simulink model "IEEE39bus"  (Simulink 8.5)
settings: Solver=ode3  SolverMode=SingleTasking  StartTime=0.0  StopTime=50  FixedStep=Ts  RelTol=1e-3
PostLoadFcn:
  | Ts=25e-6; IEEE39BusLineLength;
  | vNomHV = 345E3;fNom=50;load('Dynamicload.mat');
InitFcn:
  | Ts=25e-6; IEEE39BusLineLength;
  | vNomHV = 345E3;fNom=50;load('Dynamicload.mat');
undefined symbols (not defined in the file): D1, Delta, load15, load16, load18, load20, load21, load23, load24, load25, load26, load27, load28, load29, load3, load39, load4, load7, load8, TL_10_11_len, TL_10_13_len, TL_13_14_len, TL_14_15_len, TL_15_16_len, TL_16_17_len, TL_16_19_len, TL_16_21_len, TL_16_24_len, TL_17_18_len, TL_17_27_len, TL_1_2_len, TL_1_39_len, TL_21_22_len, TL_22_23_len, TL_24_23_len, TL_25_26_len, TL_26_27_len, TL_26_28_len, TL_26_29_len, TL_28_29_len, TL_2_25_len, TL_2_2_len, TL_3_18_len, TL_3_4_len, TL_4_14_len, TL_4_5_len, TL_5_6_len, TL_5_8_len, TL_6_11_len, TL_6_7_len, TL_7_8_len, TL_8_9_len, TL_9_39_len
libraries: powerlib x175, op_dpl_lib x34, rtlab x14, sps_avr x9, powerlib_extras x2, artemis x1, powerlib_meascontrol x1
(part 1 of 5)
settings Model: ARTEMISmethode_block_infos=$$__separator__$$IEEE39bus/ARTEMIS Guide$$__separator__$$  Creator=Admin  LastModifiedBy=Administrator
settings OptimizationCC: BlockReduction=off  OptimizeBlockIOStorage=off  BufferReuse=off  GlobalBufferReuse=off  ExpressionFolding=off  LocalBlockOutputs=off
settings DebuggingCC: SolverPrmCheckMsg=warning  FcnCallInpInsideContextMsg=EnableAllAsWarning  UnconnectedInputMsg=none  UnconnectedOutputMsg=none  UnconnectedLineMsg=none

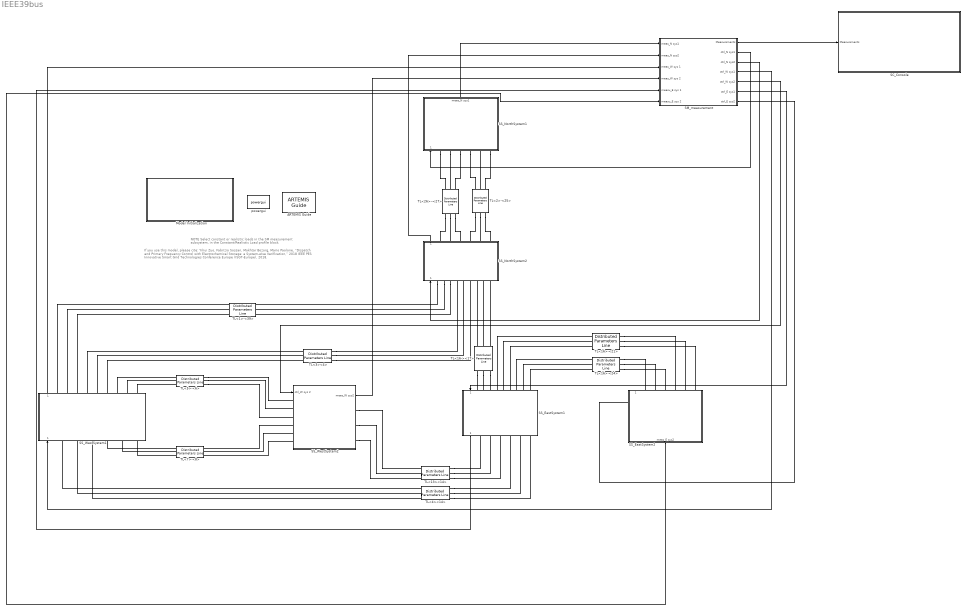
== system IEEE39bus ==
  note: If you use this model, please cite:
      | Yihui Zuo, Fabrizio Sossan, Mokhtar Bozorg, Mario Paolone,
      | “Dispatch and Primary Frequency Control with Electrochemical Storage: a System-wise Verification,”
      | 2018 IEEE PES Innovative Smart Grid Technologies Conference Europe (ISGT-Europe), 2018.
  note: NOTE
      | Select constant or realistic loads in the SM measurement
      | subsystem, in the Constant/Realistic Load profile block.
  ARTEMIS Guide : artemis/ARTEMIS/ARTEMIS Guide  Tag=FTSSmethode_opal_4hx0r99  Description=5.0_z1  lock=on  Ts=Ts  opt=art5  dyna=off  nb_perm=4  RT_fullcomp=off  ssn=on  ssn_itvc=off  ssn_ivic=off  ssn_ext=off  ssn_solver=Art5  ssn_impulse=off  ssn_quasimpulse=off  ssn_impulse_loop=2  paraExtinctionThy=off  Thy_Impulse=on  dtc=Off  dtc_opt=normal  ao=on  simtype=off  ct_mac=off  lin_mov=off  lsp=[0.001 2]  spike_skip=Disabled  dtc_extra=1  dtc_sws=normal  dtc_pied=0.5  SPSRulesBlock=SPSRules  tre=on  ctmm=off  LF=off  dpl_type=ARTEMiS DPL  rlc_type=off  custom_type=off  para=on  ssn_ImpulseLoopBlockedStateUpdate=2  ssn_mov_iter_number=5  ssn_switch_iter_number=5  ssn_nib_type_verify=on  ssn_use_lu=on  ssn_use_ldlt=off
  Model Initialization : Subsystem  AncestorBlock=artemis/Tools /Misc/Model Initialization  mask(Model Functions){InitFcnX=|, prel=off, posl=on, inif=on, strf=off}
      mask InitFcnX=|
      | Ts=25e-6; IEEE39BusLineLength;
      | vNomHV = 345E3;fNom=50;load('Dynamicload.mat');
      mask prompts: InitFcnX "Initialisation"; prel "Preload Function"; posl "PostLoad Function"; inif "InitFcn"; strf "StartFcn"
      mask init:
      | currentBlock = gcb;
      | root = bdroot(currentBlock);
      | 
      | if ~strcmp(get_param(root,'BlockDiagramType'),'library')
      |     if prel==1
      |         set_param(root, 'PreLoadFcn', InitFcnX);
      |     else
      |         set_param(root, 'PreLoadFcn', '');
      |     end
      |     if inif==1
      |         set_param(root, 'InitFcn', InitFcnX);
      |     else
      |         set_param(root, 'InitFcn', '');
      |     end
      |     if strf==1
      |         set_param(root, 'StartFcn', InitFcnX);
      |     else
      |         set_param(root, 'StartFcn', '');
      |     end
      |     if posl==1
      |         set_param(root, 'PostLoadFcn', InitFcnX);
      |     else
      |         set_param(root, 'PostLoadFcn', '');
      |     end
      | end
      | 
      | pos = get_param(currentBlock, 'Position');
      | width = pos(3) - pos(1); height = pos(4) - pos(2);
      | txt = [ upper(root) '\n' '- InitFcn. . . . . '  get_param(root, 'InitFcn') ];
      settings: CopyFcn=set_param(gcb,'LinkStatus','inactive')
      mask Display: text(5, height*0.5, txt, 'horizontalAlignment', 'left', 'verticalAlignment', 'middle') ;
  SC_Console : Subsystem
  SM_measurement : Subsystem
  SS_EastSystem1 : Subsystem
      mask Display: disp('Eastsystem 1')
  SS_EastSystem2 : Subsystem
      mask Display: disp('Eastsystem 2')
  SS_NorthSystem1 : Subsystem
      mask Display: disp('Northsystem 1')
  SS_NorthSystem2 : Subsystem
      mask Display: disp('Northsystem 2')
  SS_WestSystem1 : Subsystem
      mask Display: disp('WestSystem 1')
  SS_WestSystem2 : Subsystem
      mask Display: disp('Westsystem 2')
  TL<13><14> : op_dpl_lib/Distributed Parameters Line  SimulationMode=ARTEMIS model  Phases=3  Frequency=50  Resistance=[1.071 4.285]/TL_13_14_len  Inductance="[0.032  0.095]/TL_13_14_len"  Capacitance=[0.384e-6 0.175e-6]/TL_13_14_len  Length=TL_13_14_len  Measurements=None
  TL<16-><17> : op_dpl_lib/Distributed Parameters Line  SimulationMode=ARTEMIS model  Phases=3  Frequency=50  Resistance=[0.8332 3.33]/TL_16_17_len  Inductance="[0.028  0.084]/TL_16_17_len"  Capacitance=[0.299e-6 0.136e-6]/TL_16_17_len  Length=TL_16_17_len  Measurements=None
  TL<16>-<21> : op_dpl_lib/Distributed Parameters Line  SimulationMode=ARTEMIS model  Phases=3  Frequency=50  Resistance=[0.9522 3.809]/TL_16_21_len  Inductance="[0.043  0.128]/TL_16_21_len"  Capacitance=[0.568e-6 0.258e-6]/TL_16_21_len  Length=TL_16_21_len  Measurements=None
  TL<16>-<24> : op_dpl_lib/Distributed Parameters Line  SimulationMode=ARTEMIS model  Phases=3  Frequency=50  Resistance=[0.357 1.428]/TL_16_24_len  Inductance="[0.019  0.056]/TL_16_24_len"  Capacitance=[0.152e-6 0.069e-6]/TL_16_24_len  Length=TL_16_24_len  Measurements=None
  TL<1>-<39> : op_dpl_lib/Distributed Parameters Line  SimulationMode=ARTEMIS model  Phases=3  Frequency=50  Resistance=[1.19 4.76]/TL_1_39_len  Inductance="[0.079  0.237]/TL_1_39_len"  Capacitance=[1.67e-6 0.7599e-6]/TL_1_39_len  Length=TL_1_39_len  Measurements=None
  TL<26>--<27> : op_dpl_lib/Distributed Parameters Line  SimulationMode=ARTEMIS model  Phases=3  Frequency=50  Resistance=[1.666 6.665]/TL_26_27_len  Inductance="[0.046  0.139]/TL_26_27_len"  Capacitance=[0.534e-6 0.243e-6]/TL_26_27_len  Length=TL_26_27_len  Measurements=None
  TL<2>-<25> : op_dpl_lib/Distributed Parameters Line  SimulationMode=ARTEMIS model  Phases=3  Frequency=50  Resistance=[8.33 33.3]/TL_2_25_len  Inductance="[0.027  0.082]/TL_2_25_len"  Capacitance=[0.325e-6 0.148e-6]/TL_2_25_len  Length=TL_2_25_len  Measurements=None
  TL<3><4> : op_dpl_lib/Distributed Parameters Line  SimulationMode=ARTEMIS model  Phases=3  Frequency=50  Resistance=[1.547 6.18]/TL_3_4_len  Inductance="[0.067  0.208]/TL_3_4_len"  Capacitance=[0.493e-6 0.224e-6]/TL_3_4_len  Length=TL_3_4_len  Measurements=None
  TL<4><14> : op_dpl_lib/Distributed Parameters Line  SimulationMode=ARTEMIS model  Phases=3  Frequency=50  Resistance=[0.9522 3.808]/TL_4_14_len  Inductance="[0.041  0.1223]/TL_4_14_len"  Capacitance=[0.308e-6 0.14e-6]/TL_4_14_len  Length=TL_4_14_len  Measurements=None
  TL<5>-<6> : op_dpl_lib/Distributed Parameters Line  SimulationMode=ARTEMIS model  Phases=3  Frequency=50  Resistance=[0.476 1.904]/TL_5_6_len  Inductance=[0.014 0.04]/TL_5_6_len  Capacitance=[0.162e-6 0.074e-6]/TL_5_6_len  Length=TL_5_6_len  Measurements=None
  TL<7>-<8> : op_dpl_lib/Distributed Parameters Line  SimulationMode=ARTEMIS model  Phases=3  Frequency=50  Resistance=[0.476 1.904]/TL_7_8_len  Inductance="[0.015  0.044]/TL_7_8_len"  Capacitance=[0.174e-6 0.079e-6]/TL_7_8_len  Length=TL_7_8_len  Measurements=None
  powergui : powerlib/powergui  SimulationMode=Discrete  SolverType=Tustin  SampleTime=Ts  frequency=60  SPID=off  DisableSnubberDevices=off  DisableRonSwitches=off  DisableVfSwitches=off  SwTol=0  DisplayEquations=off  Interpol=off  methode=off  Ts=0  FunctionMessages=off  echomessages=off  HookPort=off  EnableUseOfTLC=off  x0status=steady  frequencyindice=0  Pbase=100e6  ErrMax=0.0001  Iterations=50  UnitsV=kV  UnitsW=MW  buscounter=0  RestoreLinks=warning  ResistiveCurrentMeasurement=off  Frange=[0:2:500]  Ylog=off  Xlog=on  ShowGrid=off  save=off  variable=ZData  structure=0  ZoomFFT=on  StartTime=0.0  cycles=1  DisplayStyle=1  fundamental=60  FreqAxis=off  MaxFrequency=1000  frequencyindicesteady=1  RmsSteady=2  display=off
  wires:
  SM_measurement/1(Measurements) -> SC_Console/1(Measurements)
  SM_measurement/5(ctrl_W sys2) -> SS_WestSystem2/1(ctrl_W sys 2)
  SM_measurement/6(ctrl_E sys1) -> SS_EastSystem1/1(ctrl_E sys1)
  SM_measurement/4(ctrl_W sys1) -> SS_WestSystem1/1(ctrl_W sys 1)
  SS_NorthSystem1/1(meas_N sys1) -> SM_measurement/1(meas_N sys1)
  SS_NorthSystem2/1(meas_N sys2) -> SM_measurement/2(" meas_N sys2")
  SS_EastSystem2/1(meas_E sys2) -> SM_measurement/6(measu_E sys 2)
  SS_EastSystem1/1(meas_E sys1) -> SM_measurement/5(measu_E sys 1)
  SS_WestSystem1/1(meas_W sys1) -> SM_measurement/3("meas_W sys 1  ")
  SS_WestSystem2/1(meas_W sys2) -> SM_measurement/4(" meas_W sys 2  ")
  SM_measurement/7(ctrl_E sys2) -> SS_EastSystem2/1(ctrl_E sys2)
  SM_measurement/3(ctrl_N sys2) -> SS_NorthSystem2/1(ctrl_N sys2)
  SM_measurement/2(ctrl_N sys1) -> SS_NorthSystem1/1(ctrl_N sys1)
  connections:
  SS_WestSystem1/RConn1 -- TL<1>-<39>/LConn1
  SS_WestSystem1/RConn2 -- TL<1>-<39>/LConn2
  SS_WestSystem1/RConn3 -- TL<1>-<39>/LConn3
  TL<3><4>/LConn1 -- SS_WestSystem1/RConn4
  TL<3><4>/LConn2 -- SS_WestSystem1/RConn5
  TL<3><4>/LConn3 -- SS_WestSystem1/RConn6
  TL<16-><17>/LConn2 -- SS_EastSystem1/LConn2
  TL<16-><17>/LConn1 -- SS_EastSystem1/LConn1
  TL<16-><17>/LConn3 -- SS_EastSystem1/LConn3
  TL<13><14>/RConn1 -- SS_EastSystem1/RConn1
  TL<13><14>/RConn2 -- SS_EastSystem1/RConn2
  TL<13><14>/RConn3 -- SS_EastSystem1/RConn3
  TL<4><14>/RConn1 -- SS_EastSystem1/RConn4
  TL<4><14>/RConn2 -- SS_EastSystem1/RConn5
  TL<4><14>/RConn3 -- SS_EastSystem1/RConn6
  SS_NorthSystem2/LConn1 -- TL<1>-<39>/RConn1
  SS_NorthSystem2/LConn2 -- TL<1>-<39>/RConn2
  SS_NorthSystem2/LConn3 -- TL<1>-<39>/RConn3
  TL<3><4>/RConn1 -- SS_NorthSystem2/LConn4
  TL<3><4>/RConn2 -- SS_NorthSystem2/LConn5
  TL<3><4>/RConn3 -- SS_NorthSystem2/LConn6
  TL<4><14>/LConn1 -- SS_WestSystem1/LConn1
  TL<4><14>/LConn2 -- SS_WestSystem1/LConn2
  TL<4><14>/LConn3 -- SS_WestSystem1/LConn3
  TL<16-><17>/RConn1 -- SS_NorthSystem2/LConn7
  TL<16-><17>/RConn2 -- SS_NorthSystem2/LConn8
  TL<16-><17>/RConn3 -- SS_NorthSystem2/LConn9
  SS_NorthSystem1/LConn2 -- TL<26>--<27>/LConn2
  TL<26>--<27>/RConn2 -- SS_NorthSystem2/RConn2
  TL<2>-<25>/LConn2 -- SS_NorthSystem1/LConn5
  TL<2>-<25>/RConn2 -- SS_NorthSystem2/RConn5
  SS_NorthSystem1/LConn6 -- TL<2>-<25>/LConn3
  SS_NorthSystem1/LConn4 -- TL<2>-<25>/LConn1
  SS_NorthSystem1/LConn3 -- TL<26>--<27>/LConn3
  SS_NorthSystem1/LConn1 -- TL<26>--<27>/LConn1
  TL<26>--<27>/RConn1 -- SS_NorthSystem2/RConn1
  TL<26>--<27>/RConn3 -- SS_NorthSystem2/RConn3
  TL<2>-<25>/RConn3 -- SS_NorthSystem2/RConn6
  TL<2>-<25>/RConn1 -- SS_NorthSystem2/RConn4
  TL<16>-<24>/LConn1 -- SS_EastSystem1/LConn7
  TL<16>-<24>/LConn2 -- SS_EastSystem1/LConn8
  TL<16>-<24>/LConn3 -- SS_EastSystem1/LConn9
  TL<16>-<24>/RConn3 -- SS_EastSystem2/LConn3
  TL<16>-<24>/RConn2 -- SS_EastSystem2/LConn2
  TL<16>-<24>/RConn1 -- SS_EastSystem2/LConn1
  SS_EastSystem1/LConn4 -- TL<16>-<21>/LConn1
  SS_EastSystem1/LConn5 -- TL<16>-<21>/LConn2
  SS_EastSystem1/LConn6 -- TL<16>-<21>/LConn3
  TL<16>-<21>/RConn1 -- SS_EastSystem2/LConn4
  TL<16>-<21>/RConn2 -- SS_EastSystem2/LConn5
  TL<16>-<21>/RConn3 -- SS_EastSystem2/LConn6
  SS_WestSystem2/RConn1 -- TL<13><14>/LConn1
  SS_WestSystem2/RConn2 -- TL<13><14>/LConn2
  SS_WestSystem2/RConn3 -- TL<13><14>/LConn3
  TL<5>-<6>/LConn1 -- SS_WestSystem1/RConn7
  TL<5>-<6>/LConn2 -- SS_WestSystem1/RConn8
  TL<5>-<6>/LConn3 -- SS_WestSystem1/RConn9
  TL<5>-<6>/RConn1 -- SS_WestSystem2/LConn1
  TL<5>-<6>/RConn2 -- SS_WestSystem2/LConn2
  TL<5>-<6>/RConn3 -- SS_WestSystem2/LConn3
  SS_WestSystem2/LConn4 -- TL<7>-<8>/RConn1
  SS_WestSystem2/LConn5 -- TL<7>-<8>/RConn2
  SS_WestSystem2/LConn6 -- TL<7>-<8>/RConn3
  TL<7>-<8>/LConn1 -- SS_WestSystem1/LConn4
  TL<7>-<8>/LConn2 -- SS_WestSystem1/LConn5
  TL<7>-<8>/LConn3 -- SS_WestSystem1/LConn6

== system IEEE39bus/Model Initialization ==

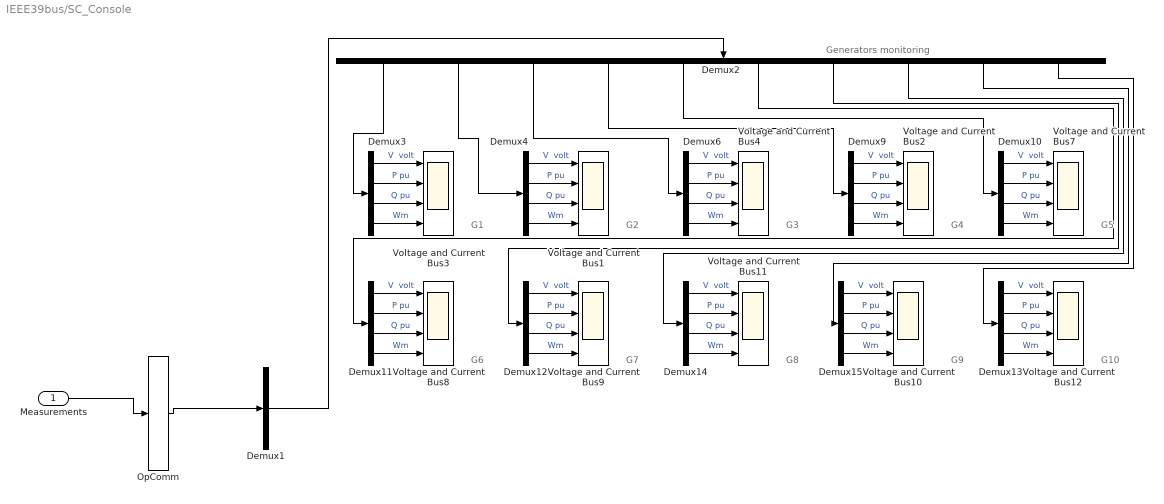
== system IEEE39bus/SC_Console ==
  note: G10
  note: G9
  note: G8
  note: G7
  note: G6
  note: G5
  note: G4
  note: G3
  note: G2
  note: G1
  note: Generators monitoring
  Measurements : Inport
  Demux1 : Demux  Outputs=[60 ]
  Demux{3..4,6,9..15} (10 alike) : Demux  Outputs=[3 1 1 1]
  Demux2 : Demux  Outputs=[6 6 6 6 6 6 6 6 6 6]
  OpComm : rtlab/OpComm  nbport=1  groupe_acq=1  subsys_rate=30*Ts  st=0  Synchronization=on  Interpolation=on  Threshold=1.0  Missed_Data=off  Sim_Time=off  Samples=off  dynSigOut=off  from_console=0  warning_done=off  writeOpCommFile=off  Offset=off
  Voltage and Current Bus{1..4,7..12} (10 alike) : Scope  NumInputPorts=4
      Voltage and Current Bus1 settings: TimeRange=0.24  YMin=-20000~0.715~0.2785~0.99755  YMax=20000~0.723~0.2835~0.99763  SaveName=mach  MaxDataPoints=15000
      Voltage and Current Bus10 settings: TimeRange=0.24  YMin=-20000~0.576~0.052~0.99807  YMax=20000~0.584~0.063~0.99816  SaveName=mach9  MaxDataPoints=15000
      Voltage and Current Bus11 settings: TimeRange=0.24  YMin=-20000~0.599~0.017~1.00427  YMax=20000~0.605~0.022~1.00438  SaveName=mach10  MaxDataPoints=15000
      Voltage and Current Bus12 settings: TimeRange=0.24  YMin=-20000~0.336~0.015~0.99933  YMax=20000~0.346~0.022~0.99942  SaveName=mach11  MaxDataPoints=15000
      Voltage and Current Bus2 settings: TimeRange=0.24  YMin=-20000~0.556~-0.038~0.99875  YMax=20000~0.563~-0.0335~0.99905  SaveName=mach2  MaxDataPoints=15000
      Voltage and Current Bus3 settings: TimeRange=22.5285  YMin=-20000~0.45~0.07~0.99775  YMax=20000~0.55~0.145~1.00125  SaveName=mach1  MaxDataPoints=15000
      Voltage and Current Bus4 settings: TimeRange=0.24  YMin=-20000~0.51~0.2~0.99932  YMax=20000~0.545~0.24~0.9994  SaveName=mach3  MaxDataPoints=15000
      Voltage and Current Bus7 settings: TimeRange=0.24  YMin=-20000~0.753~0.1225~0.982477  YMax=20000~0.7575~0.127~0.982495  SaveName=mach6  MaxDataPoints=15000
      Voltage and Current Bus8 settings: TimeRange=0.24  YMin=-20000~0.5~0.02~0.9963  YMax=20000~0.61~0.13~0.9973  SaveName=mach7  MaxDataPoints=15000
      Voltage and Current Bus9 settings: TimeRange=0.24  YMin=-20000~0.4425~-0.053~0.9993  YMax=20000~0.465~-0.046~0.99955  SaveName=mach8  MaxDataPoints=15000
  wires:
  Demux1/1 -> Demux2/1
  Demux2/10 -> Demux13/1
  Demux2/9 -> Demux15/1
  Demux2/8 -> Demux14/1
  Demux2/7 -> Demux12/1
  Demux2/6 -> Demux11/1
  Demux2/5 -> Demux10/1
  Demux2/4 -> Demux9/1
  Demux2/3 -> Demux6/1
  Demux2/2 -> Demux4/1
  Demux2/1 -> Demux3/1
  OpComm/1 -> Demux1/1
  Measurements/1 -> OpComm/1
  Demux3/1 -> Voltage and Current Bus3/1  "V  volt"
  Demux3/3 -> Voltage and Current Bus3/3  "Q pu"
  Demux3/4 -> Voltage and Current Bus3/4  "Wm"
  Demux3/2 -> Voltage and Current Bus3/2  "P pu"
  Demux4/1 -> Voltage and Current Bus1/1  "V  volt"
  Demux4/3 -> Voltage and Current Bus1/3  "Q pu"
  Demux4/4 -> Voltage and Current Bus1/4  "Wm"
  Demux4/2 -> Voltage and Current Bus1/2  "P pu"
  Demux6/1 -> Voltage and Current Bus4/1  "V  volt"
  Demux6/3 -> Voltage and Current Bus4/3  "Q pu"
  Demux6/4 -> Voltage and Current Bus4/4  "Wm"
  Demux6/2 -> Voltage and Current Bus4/2  "P pu"
  Demux9/1 -> Voltage and Current Bus2/1  "V  volt"
  Demux9/3 -> Voltage and Current Bus2/3  "Q pu"
  Demux9/4 -> Voltage and Current Bus2/4  "Wm"
  Demux9/2 -> Voltage and Current Bus2/2  "P pu"
  Demux10/1 -> Voltage and Current Bus7/1  "V  volt"
  Demux10/3 -> Voltage and Current Bus7/3  "Q pu"
  Demux10/4 -> Voltage and Current Bus7/4  "Wm"
  Demux10/2 -> Voltage and Current Bus7/2  "P pu"
  Demux11/1 -> Voltage and Current Bus8/1  "V  volt"
  Demux11/3 -> Voltage and Current Bus8/3  "Q pu"
  Demux11/4 -> Voltage and Current Bus8/4  "Wm"
  Demux11/2 -> Voltage and Current Bus8/2  "P pu"
  Demux12/1 -> Voltage and Current Bus9/1  "V  volt"
  Demux12/3 -> Voltage and Current Bus9/3  "Q pu"
  Demux12/4 -> Voltage and Current Bus9/4  "Wm"
  Demux12/2 -> Voltage and Current Bus9/2  "P pu"
  Demux14/1 -> Voltage and Current Bus11/1  "V  volt"
  Demux14/3 -> Voltage and Current Bus11/3  "Q pu"
  Demux14/4 -> Voltage and Current Bus11/4  "Wm"
  Demux14/2 -> Voltage and Current Bus11/2  "P pu"
  Demux15/1 -> Voltage and Current Bus10/1  "V  volt"
  Demux15/3 -> Voltage and Current Bus10/3  "Q pu"
  Demux15/4 -> Voltage and Current Bus10/4  "Wm"
  Demux15/2 -> Voltage and Current Bus10/2  "P pu"
  Demux13/1 -> Voltage and Current Bus12/1  "V  volt"
  Demux13/3 -> Voltage and Current Bus12/3  "Q pu"
  Demux13/4 -> Voltage and Current Bus12/4  "Wm"
  Demux13/2 -> Voltage and Current Bus12/2  "P pu"

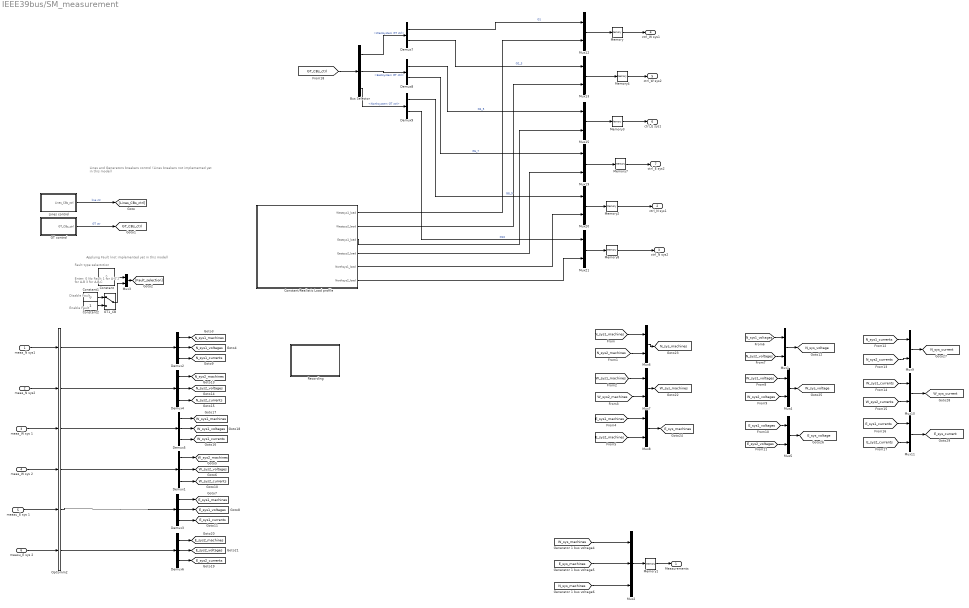
== system IEEE39bus/SM_measurement ==
  note: Enable Fault
  note: Disable Fault
  note: Enter:  0 No Fault
      |          1 for A-G
      |          2 for A-B
      |              3 for A-B-C
  note: Fault type selectction
  note: Applying Fault
      | (not implemented yet in this model)
  note: Lines and Generators breakers control
      | (Lines breakers not implemented yet in this model)
  meas_N sys1 : Inport
  " meas_N sys2" : Inport  Port=2
  "meas_W sys 1  " : Inport  Port=3
  " meas_W sys 2  " : Inport  Port=4
  measu_E sys 1 : Inport  Port=5
  measu_E sys 2 : Inport  Port=6
  Bus Selector : BusSelector  OutputSignals=Westsystem GT ctrl,Eastsystem GT ctrl,Northsystem GT ctrl
  Constant : Constant  Value=2
  Constant/Realistic Load profile : Subsystem  SystemSampleTime=20e-3  mask{Loadselect=Constant Load}
      mask init:
      | if (Loadselect == 1)
      |     mode = 0;
      | else 
      |         mode = 1; 
      | end
      mask TypeOptions Loadselect: Constant Load | Realistic Load
      mask Display: disp('Load Profile \n Constant / Realistic')
  Constant1 : Constant  Value=0
  Constant2 : Constant
  Demux1 : Demux  Outputs=[12 18 18]
  Demux2 : Demux  Outputs=[12 12 12]
  Demux3 : Demux  Outputs=[12 15 15]
  Demux4 : Demux  Outputs=[6 18 18]
  Demux5 : Demux  Outputs=[6 15 15]
  Demux6 : Demux  Outputs=[12 12 12]
  Demux7 : Demux  Outputs=[1 2]
  Demux8 : Demux  Outputs=[2 2]
  Demux9 : Demux  Outputs=[2 1]
  GT control : Subsystem
  GT1_CB : ManualSwitch
  Lines control : Subsystem
  Memory{,1..4,7..8} (7 alike) : Memory
  Mux{1,3..13,15,19..21} (16 alike) : Mux  Inputs=2
  Mux2 : Mux  Inputs=3
  OpComm2 : rtlab/OpComm  nbport=6  groupe_acq=1  subsys_rate=0  st=Ts  Synchronization=on  Interpolation=on  Threshold=1.0  Missed_Data=off  Sim_Time=off  Samples=off  dynSigOut=off  from_console=0  warning_done=off  writeOpCommFile=off  Offset=off
  Recording : Subsystem
  Measurements : Outport
  ctrl_N sys1 : Outport  Port=2
  ctrl_N sys2 : Outport  Port=3
  ctrl_W sys1 : Outport  Port=4
  ctrl_W sys2 : Outport  Port=5
  ctrl_E sys1 : Outport  Port=6
  ctrl_E sys2 : Outport  Port=7
  tag scope: E_sys1_currents=global, E_sys1_machines=global, E_sys1_voltages=global, E_sys2_currents=global, E_sys2_machines=global, E_sys2_voltages=global, E_sys_current=global, E_sys_machines=global, E_sys_voltage=global, GT_CBs_ctrl=global, N_sys1_currents=global, N_sys1_machines=global, N_sys1_voltages=global, N_sys2_currents=global, N_sys2_machines=global, N_sys2_voltages=global, N_sys_current=global, N_sys_machines=global, N_sys_voltage=global, W_sys1_currents=global, W_sys1_machines=global, W_sys1_voltages=global, W_sys2_currents=global, W_sys2_machines=global, W_sys2_voltages=global, W_sys_current=global, W_sys_machines=global, W_sys_voltage=global
  wires:
  Demux3/2 -> [E_sys1_voltages]
  Demux1/2 -> [W_sys2_voltages]
  Demux2/2 -> [N_sys1_voltages]
  Memory1/1 -> Measurements/1
  [N_sys_machines] -> Mux2/3
  [E_sys_machines] -> Mux2/2
  [W_sys_machines] -> Mux2/1
  Demux3/1 -> [E_sys1_machines]
  Demux1/1 -> [W_sys2_machines]
  " meas_W sys 2  "/1 -> OpComm2/4
  " meas_N sys2"/1 -> OpComm2/2
  Mux2/1 -> Memory1/1
  OpComm2/1 -> Demux2/1
  Demux2/1 -> [N_sys1_machines]
  Demux2/3 -> [N_sys1_currents]
  Demux1/3 -> [W_sys2_currents]
  Demux3/3 -> [E_sys1_currents]
  Constant/1 -> Mux3/1
  GT1_CB/1 -> Mux3/2
  Constant1/1 -> GT1_CB/1
  Constant2/1 -> GT1_CB/2
  GT control/1(GT_CBs_ctrl) -> [GT_CBs_ctrl]  "GT ctr"
  Lines control/1(Lines_CBs_ctrl) -> [Lines_CBs_ctrl]  "line ctr"
  Mux3/1 -> [Fault_selection]
  meas_N sys1/1 -> OpComm2/1
  "meas_W sys 1  "/1 -> OpComm2/3
  measu_E sys 1/1 -> OpComm2/5
  measu_E sys 2/1 -> OpComm2/6
  Demux4/2 -> [N_sys2_voltages]
  Demux4/1 -> [N_sys2_machines]
  Demux4/3 -> [N_sys2_currents]
  OpComm2/2 -> Demux4/1
  OpComm2/4 -> Demux1/1
  Demux5/2 -> [W_sys1_voltages]
  Demux5/1 -> [W_sys1_machines]
  Demux5/3 -> [W_sys1_currents]
  OpComm2/3 -> Demux5/1
  OpComm2/5 -> Demux3/1
  Demux6/2 -> [E_sys2_voltages]
  Demux6/1 -> [E_sys2_machines]
  Demux6/3 -> [E_sys2_currents]
  OpComm2/6 -> Demux6/1
  [N_sys2_machines] -> Mux6/2
  [N_sys1_machines] -> Mux6/1
  Mux6/1 -> [N_sys_machines]
  [W_sys1_machines] -> Mux7/1
  [W_sys2_machines] -> Mux7/2
  Mux7/1 -> [W_sys_machines]
  [E_sys1_machines] -> Mux8/1
  [E_sys2_machines] -> Mux8/2
  Mux8/1 -> [E_sys_machines]
  [N_sys1_voltages] -> Mux1/1
  [N_sys2_voltages] -> Mux1/2
  [W_sys1_voltages] -> Mux4/1
  [W_sys2_voltages] -> Mux4/2
  [E_sys1_voltages] -> Mux5/1
  [E_sys2_voltages] -> Mux5/2
  Mux1/1 -> [N_sys_voltage]
  Mux4/1 -> [W_sys_voltage]
  Mux5/1 -> [E_sys_voltage]
  [N_sys1_currents] -> Mux9/1
  [N_sys2_currents] -> Mux9/2
  [W_sys1_currents] -> Mux10/1
  [W_sys2_currents] -> Mux10/2
  [E_sys1_currents] -> Mux11/1
  [E_sys2_currents] -> Mux11/2
  Mux9/1 -> [N_sys_current]
  Mux10/1 -> [W_sys_current]
  Mux11/1 -> [E_sys_current]
  Memory2/1 -> ctrl_N sys1/1
  Memory3/1 -> ctrl_E sys1/1
  Memory/1 -> ctrl_W sys1/1
  Constant/Realistic Load profile/1(Westsys1_load) -> Mux12/2
  Constant/Realistic Load profile/2(Westsys2_laod) -> Mux13/2
  Memory4/1 -> ctrl_W sys2/1
  Constant/Realistic Load profile/3(Eastsys1_load) -> Mux15/2
  Constant/Realistic Load profile/4(Eastsys2_load) -> Mux19/2
  Memory7/1 -> ctrl_E sys2/1
  Constant/Realistic Load profile/5(Northsys1_load) -> Mux20/2
  Constant/Realistic Load profile/6(Northsys2_load) -> Mux21/2
  Memory8/1 -> ctrl_N sys2/1
  Mux20/1 -> Memory2/1
  [GT_CBs_ctrl] -> Bus Selector/1
  Bus Selector/2 -> Demux8/1  "<Eastsystem GT ctrl>"
  Bus Selector/1 -> Demux7/1  "<Westsystem GT ctrl>"
  Bus Selector/3 -> Demux9/1  "<Northsystem GT ctrl>"
  Demux7/1 -> Mux12/1  "G1"
  Mux12/1 -> Memory/1
  Demux7/2 -> Mux13/1  "G2_3"
  Mux13/1 -> Memory4/1
  Demux8/1 -> Mux15/1  "G4_5"
  Demux8/2 -> Mux19/1  "G6_7"
  Mux15/1 -> Memory3/1
  Mux19/1 -> Memory7/1
  Demux9/1 -> Mux20/1  "G8_9"
  Demux9/2 -> Mux21/1  "G10"
  Mux21/1 -> Memory8/1

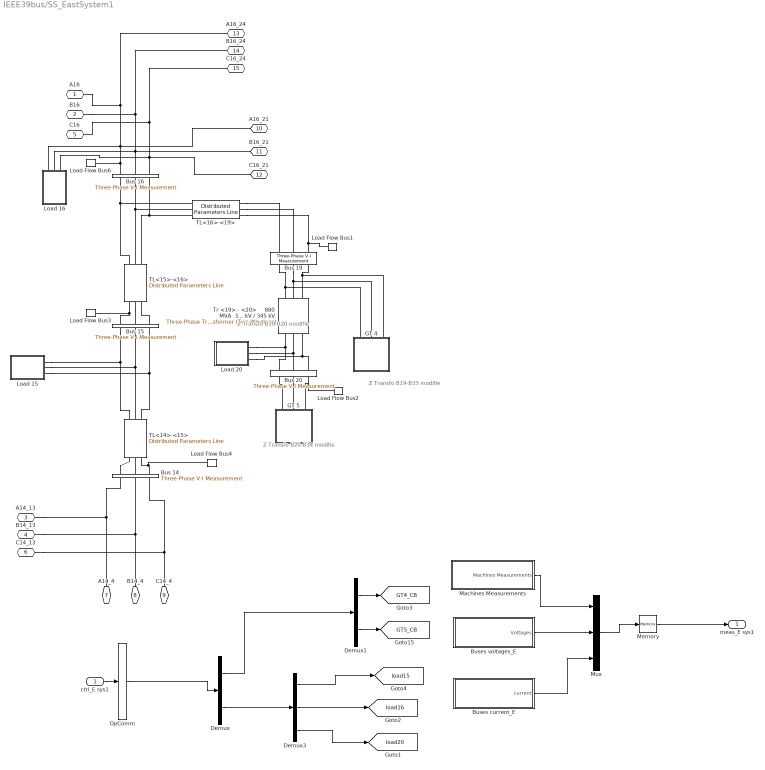
== system IEEE39bus/SS_EastSystem1 ==
  note: Z Transfo B19-B20 modifie
  note: Z Transfo B20-B34 modifie
  note: Z Transfo B19-B33 modifie
  ctrl_E sys1 : Inport
  Bus 14 : powerlib/Measurements/Three-Phase V-I Measurement  VoltageMeasurement=phase-to-ground  SetLabelV=on  LabelV=V_bus_14  Vpu=off  VpuLL=off  CurrentMeasurement=yes  SetLabelI=on  LabelI=I_bus_14  Ipu=off  Pbase=100e6  Vbase=230e3  OutputType=Complex  PhasorSimulation=off  PSBequivalent=0
  Bus 15 : powerlib/Measurements/Three-Phase V-I Measurement  VoltageMeasurement=phase-to-ground  SetLabelV=on  LabelV=V_bus_15  Vpu=off  VpuLL=off  CurrentMeasurement=yes  SetLabelI=on  LabelI=I_bus_15  Ipu=off  Pbase=100e6  Vbase=230e3  OutputType=Complex  PhasorSimulation=off  PSBequivalent=0
  Bus 16 : powerlib/Measurements/Three-Phase V-I Measurement  VoltageMeasurement=phase-to-ground  SetLabelV=on  LabelV=V_bus_16  Vpu=off  VpuLL=off  CurrentMeasurement=yes  SetLabelI=on  LabelI=I_bus_16  Ipu=off  Pbase=100e6  Vbase=230e3  OutputType=Complex  PhasorSimulation=off  PSBequivalent=0
  Bus 19 : powerlib/Measurements/Three-Phase V-I Measurement  VoltageMeasurement=phase-to-ground  SetLabelV=on  LabelV=V_bus_19  Vpu=off  VpuLL=off  CurrentMeasurement=yes  SetLabelI=on  LabelI=I_bus_19  Ipu=off  Pbase=100e6  Vbase=230e3  OutputType=Complex  PhasorSimulation=off  PSBequivalent=0
  Bus 20 : powerlib/Measurements/Three-Phase V-I Measurement  VoltageMeasurement=phase-to-ground  SetLabelV=on  LabelV=V_bus_20  Vpu=off  VpuLL=off  CurrentMeasurement=yes  SetLabelI=on  LabelI=I_bus_20  Ipu=off  Pbase=100e6  Vbase=230e3  OutputType=Complex  PhasorSimulation=off  PSBequivalent=0
  Buses current_E : Subsystem
  Buses voltages_E : Subsystem
  Demux : Demux  Outputs=[2 6]
  Demux1 : Demux  Outputs=2
  Demux3 : Demux  Outputs=[2 2 2]
  GT 4 : Subsystem
  GT 5 : Subsystem
  Load 15 : Subsystem
  Load 16 : Subsystem
  Load 20 : Subsystem
  Load Flow Bus1 : powerlib/Measurements/Load Flow Bus  LConnTagsString=a  ID=Bus-19  Vbase=345e+003  Vref=1  Vangle=0  VLF=1.019  angleLF=21.55
      settings: AttributesFormatString=%<ID>\n%<Vbase>V\n%<VLF>pu\n%<angleLF>deg.
  Load Flow Bus2 : powerlib/Measurements/Load Flow Bus  LConnTagsString=a  ID=Bus-20  Vbase=345e+003  Vref=1  Vangle=0  VLF=0.9613  angleLF=-10.55
      settings: AttributesFormatString=%<ID>\n%<Vbase>V\n%<VLF>pu\n%<angleLF>deg.
  Load Flow Bus3 : powerlib/Measurements/Load Flow Bus  LConnTagsString=a  ID=Bus-15  Vbase=345e+003  Vref=1  Vangle=0  VLF=0.996  angleLF=18.53
      settings: AttributesFormatString=%<ID>\n%<Vbase>V\n%<VLF>pu\n%<angleLF>deg.
  Load Flow Bus4 : powerlib/Measurements/Load Flow Bus  LConnTagsString=a  ID=Bus-14  Vbase=345e+003  Vref=1  Vangle=0  VLF=1.001  angleLF=20.12
      settings: AttributesFormatString=%<ID>\n%<Vbase>V\n%<VLF>pu\n%<angleLF>deg.
  Load Flow Bus6 : powerlib/Measurements/Load Flow Bus  LConnTagsString=a  ID=Bus-16  Vbase=345e+003  Vref=1  Vangle=0  VLF=1.007  angleLF=19.22
      settings: AttributesFormatString=%<ID>\n%<Vbase>V\n%<VLF>pu\n%<angleLF>deg.
  Machines Measurements : Subsystem
      mask Display: disp('Machines Measurements')
  Memory : Memory
  Mux : Mux  Inputs=3
  OpComm : rtlab/OpComm  nbport=1  groupe_acq=1  subsys_rate=0  st=0  Synchronization=on  Interpolation=on  Threshold=1.0  Missed_Data=off  Sim_Time=off  Samples=off  dynSigOut=off  from_console=0  warning_done=off  writeOpCommFile=off  Offset=off
  TL<14>-<15> : op_dpl_lib/Distributed Parameters Line  SimulationMode=ARTEMIS model  Phases=3  Frequency=50  Resistance=[2.142 8.57]/TL_14_15_len  Inductance="[0.069  0.206]/TL_14_15_len"  Capacitance=[0.816e-6 0.371e-6]/TL_14_15_len  Length=TL_14_15_len  Measurements=None
  TL<15>-<16> : op_dpl_lib/Distributed Parameters Line  SimulationMode=ARTEMIS model  Phases=3  Frequency=50  Resistance=[1.071 4.285]/TL_15_16_len  Inductance="[0.03  0.089]/TL_15_16_len"  Capacitance=[0.381e-6 0.173e-6]/TL_15_16_len  Length=TL_15_16_len  Measurements=None
  TL<16>-<19> : op_dpl_lib/Distributed Parameters Line  SimulationMode=ARTEMIS model  Phases=3  Frequency=50  Resistance=[1.904 7.618]/TL_16_19_len  Inductance="[0.062  0.185]/TL_16_19_len"  Capacitance=[0.677e-6 0.308e-6]/TL_16_19_len  Length=TL_16_19_len  Measurements=None
  Tr <19> - <20>     880 MVA  345 kV / 345 kV : powerlib/Elements/Three-Phase Transformer (Two Windings)  Winding1Connection=Delta (D1)  Winding2Connection=Yg  CoreType=Three single-phase transformers  SetSaturation=off  Hysteresis=off  DataFile='hysteresis'  SetInitialFlux=off  Measurements=None  UNITS=pu  NominalPower=[ 880e6 50]  Winding1="[ 345e3 0.0007*880/100/2   0.0138*880/100/2 ]"  Winding2="[ 1.06*345e3 0.0007*880/100/2   0.0138*880/100/2 ]"  Rm=500  Lm=500  L0=0.5  Saturation="[ 0,0  ;  0.005,1.2  ;  1.0,1.4 ]"  InitialFluxes=[ 0.8 , -0.8 , 0.7 ]  MoreParameters=off  BreakLoop=off  DataType=off  TransfoNumber=0
  A16 : PMIOPort  Port=1  Side=Left
  B16 : PMIOPort  Port=2  Side=Left
  A14_13 : PMIOPort  Port=3  Side=Right
  B14_13 : PMIOPort  Port=4  Side=Right
  C16 : PMIOPort  Port=5  Side=Left
  C14_13 : PMIOPort  Port=6  Side=Right
  A14_4 : PMIOPort  Port=7  Side=Right
  B14_4 : PMIOPort  Port=8  Side=Right
  C14_4 : PMIOPort  Port=9  Side=Right
  A16_21 : PMIOPort  Port=10  Side=Left
  B16_21 : PMIOPort  Port=11  Side=Left
  C16_21 : PMIOPort  Port=12  Side=Left
  A16_24 : PMIOPort  Port=13  Side=Left
  B16_24 : PMIOPort  Port=14  Side=Left
  C16_24 : PMIOPort  Port=15  Side=Left
  meas_E sys1 : Outport
  tag scope: GT4_CB=global, GT5_CB=global, load15=global, load16=global, load20=global
  wires:
  ctrl_E sys1/1 -> OpComm/1
  Machines Measurements/1(Machines Measurements) -> Mux/1
  Mux/1 -> Memory/1
  Memory/1 -> meas_E sys1/1
  Buses voltages_E/1(Voltages) -> Mux/2
  Buses current_E/1(current) -> Mux/3
  OpComm/1 -> Demux/1
  Demux/1 -> Demux1/1
  Demux1/2 -> [GT5_CB]
  Demux/2 -> Demux3/1
  Demux3/1 -> [load15]
  Demux3/2 -> [load16]
  Demux3/3 -> [load20]
  Demux1/1 -> [GT4_CB]
  connections:
  A14_4/RConn1 -- A14_13/RConn1 -- Bus 14/LConn1
  C14_4/RConn1 -- Bus 14/LConn3 -- C14_13/RConn1
  B14_4/RConn1 -- B14_13/RConn1 -- Bus 14/LConn2
  Tr <19> - <20>     880 MVA  345 kV / 345 kV/LConn3 -- Load 20/LConn3 -- Bus 20/RConn3
  Load 20/LConn2 -- Tr <19> - <20>     880 MVA  345 kV / 345 kV/LConn2 -- Bus 20/RConn2
  Load 20/LConn1 -- Tr <19> - <20>     880 MVA  345 kV / 345 kV/LConn1 -- Bus 20/RConn1
  GT 5/RConn3 -- Bus 20/LConn3 -- Load Flow Bus2/LConn1
  Bus 20/LConn2 -- GT 5/RConn2
  GT 5/RConn1 -- Bus 20/LConn1
  GT 4/RConn3 -- Tr <19> - <20>     880 MVA  345 kV / 345 kV/RConn3 -- Bus 19/LConn3
  GT 4/RConn2 -- Tr <19> - <20>     880 MVA  345 kV / 345 kV/RConn2 -- Bus 19/LConn2
  GT 4/RConn1 -- Tr <19> - <20>     880 MVA  345 kV / 345 kV/RConn1 -- Bus 19/LConn1
  C16/RConn1 -- C16_24/RConn1 -- Load 16/LConn3 -- Bus 16/RConn3 -- C16_21/RConn1
  B16/RConn1 -- B16_24/RConn1 -- Load 16/LConn2 -- B16_21/RConn1 -- Bus 16/RConn2
  Load Flow Bus6/LConn1 -- Bus 16/RConn1 -- Load 16/LConn1 -- A16_21/RConn1 -- A16_24/RConn1 -- A16/RConn1
  Bus 15/RConn3 -- TL<15>-<16>/RConn3
  TL<15>-<16>/RConn2 -- Bus 15/RConn2
  Load Flow Bus3/LConn1 -- TL<15>-<16>/RConn1 -- Bus 15/RConn1
  Bus 14/RConn3 -- Load Flow Bus4/LConn1 -- TL<14>-<15>/RConn3
  Bus 14/RConn2 -- TL<14>-<15>/RConn2
  Bus 14/RConn1 -- TL<14>-<15>/RConn1
  Bus 16/LConn1 -- TL<15>-<16>/LConn1 -- TL<16>-<19>/LConn1
  Bus 16/LConn2 -- TL<15>-<16>/LConn2 -- TL<16>-<19>/LConn2
  Bus 16/LConn3 -- TL<15>-<16>/LConn3 -- TL<16>-<19>/LConn3
  Load 15/LConn1 -- TL<14>-<15>/LConn1 -- Bus 15/LConn1
  Load 15/LConn2 -- TL<14>-<15>/LConn2 -- Bus 15/LConn2
  Bus 15/LConn3 -- TL<14>-<15>/LConn3 -- Load 15/LConn3
  TL<16>-<19>/RConn1 -- Bus 19/RConn1
  TL<16>-<19>/RConn2 -- Bus 19/RConn2
  Bus 19/RConn3 -- TL<16>-<19>/RConn3 -- Load Flow Bus1/LConn1

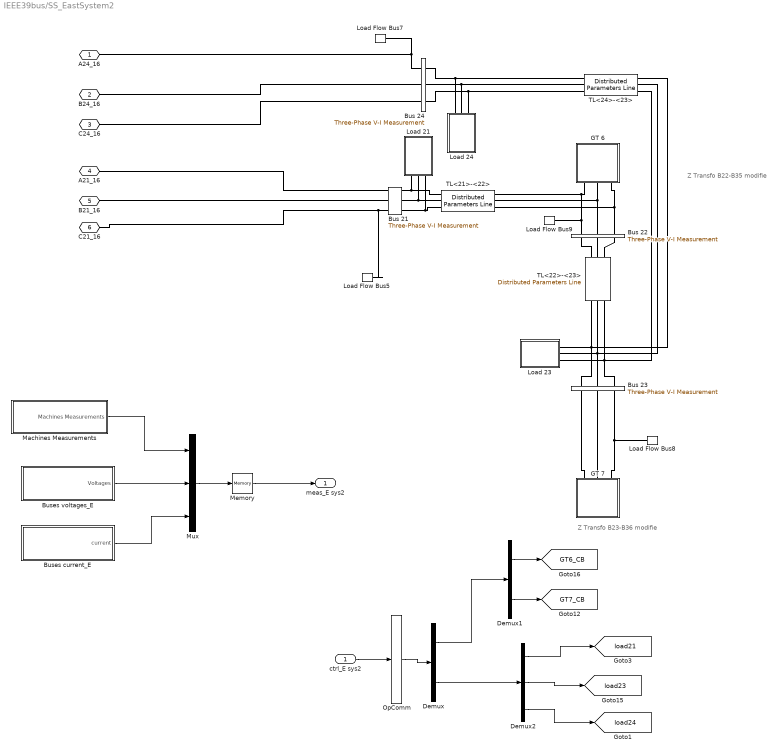
== system IEEE39bus/SS_EastSystem2 ==
  note: Z Transfo B22-B35 modifie
  note: Z Transfo B23-B36 modifie
  ctrl_E sys2 : Inport
  Bus 21 : powerlib/Measurements/Three-Phase V-I Measurement  VoltageMeasurement=phase-to-ground  SetLabelV=on  LabelV=V_bus_21  Vpu=off  VpuLL=off  CurrentMeasurement=yes  SetLabelI=on  LabelI=I_bus_21  Ipu=off  Pbase=100e6  Vbase=230e3  OutputType=Complex  PhasorSimulation=off  PSBequivalent=0
  Bus 22 : powerlib/Measurements/Three-Phase V-I Measurement  VoltageMeasurement=phase-to-ground  SetLabelV=on  LabelV=V_bus_22  Vpu=off  VpuLL=off  CurrentMeasurement=yes  SetLabelI=on  LabelI=I_bus_22  Ipu=off  Pbase=100e6  Vbase=230e3  OutputType=Complex  PhasorSimulation=off  PSBequivalent=0
  Bus 23 : powerlib/Measurements/Three-Phase V-I Measurement  VoltageMeasurement=phase-to-ground  SetLabelV=on  LabelV=V_bus_23  Vpu=off  VpuLL=off  CurrentMeasurement=yes  SetLabelI=on  LabelI=I_bus_23  Ipu=off  Pbase=100e6  Vbase=230e3  OutputType=Complex  PhasorSimulation=off  PSBequivalent=0
  Bus 24 : powerlib/Measurements/Three-Phase V-I Measurement  VoltageMeasurement=phase-to-ground  SetLabelV=on  LabelV=V_bus_24  Vpu=off  VpuLL=off  CurrentMeasurement=yes  SetLabelI=on  LabelI=I_bus_24  Ipu=off  Pbase=100e6  Vbase=230e3  OutputType=Complex  PhasorSimulation=off  PSBequivalent=0
  Buses current_E : Subsystem
  Buses voltages_E : Subsystem
  Demux : Demux  Outputs=[2 6]
  Demux1 : Demux  Outputs=2
  Demux2 : Demux  Outputs=[2 2 2]
  GT 6 : Subsystem
  GT 7 : Subsystem
  Load 21 : Subsystem
  Load 23 : Subsystem
  Load 24 : Subsystem
  Load Flow Bus5 : powerlib/Measurements/Load Flow Bus  LConnTagsString=a  ID=Bus-21  Vbase=345e+003  Vref=1  Vangle=0  VLF=1.006  angleLF=20.56
      settings: AttributesFormatString=%<ID>\n%<Vbase>V\n%<VLF>pu\n%<angleLF>deg.
  Load Flow Bus7 : powerlib/Measurements/Load Flow Bus  LConnTagsString=a  ID=Bus-24  Vbase=345e+003  Vref=1  Vangle=0  VLF=1.011  angleLF=19.08
      settings: AttributesFormatString=%<ID>\n%<Vbase>V\n%<VLF>pu\n%<angleLF>deg.
  Load Flow Bus8 : powerlib/Measurements/Load Flow Bus  LConnTagsString=a  ID=Bus-23  Vbase=345e+003  Vref=1  Vangle=0  VLF=1.012  angleLF=23.42
      settings: AttributesFormatString=%<ID>\n%<Vbase>V\n%<VLF>pu\n%<angleLF>deg.
  Load Flow Bus9 : powerlib/Measurements/Load Flow Bus  LConnTagsString=a  ID=Bus-22  Vbase=345e+003  Vref=1  Vangle=0  VLF=1.019  angleLF=23.66
      settings: AttributesFormatString=%<ID>\n%<Vbase>V\n%<VLF>pu\n%<angleLF>deg.
  Machines Measurements : Subsystem
      mask Display: disp('Machines Measurements')
  Memory : Memory
  Mux : Mux  Inputs=3
  OpComm : rtlab/OpComm  nbport=1  groupe_acq=1  subsys_rate=0  st=0  Synchronization=on  Interpolation=on  Threshold=1.0  Missed_Data=off  Sim_Time=off  Samples=off  dynSigOut=off  from_console=0  warning_done=off  writeOpCommFile=off  Offset=off
  TL<21>-<22> : op_dpl_lib/Distributed Parameters Line  SimulationMode=ARTEMIS model  Phases=3  Frequency=50  Resistance=[0.9522 3.809]/TL_21_22_len  Inductance="[0.044  0.133]/TL_21_22_len"  Capacitance=[0.572e-6 0.26e-6]/TL_21_22_len  Length=TL_21_22_len  Measurements=None
  TL<22>-<23> : op_dpl_lib/Distributed Parameters Line  SimulationMode=ARTEMIS model  Phases=3  Frequency=50  Resistance=[0.714 2.857]/TL_22_23_len  Inductance="[0.03  0.091]/TL_22_23_len"  Capacitance=[0.411e-6 0.187e-6]/TL_22_23_len  Length=TL_22_23_len  Measurements=None
  TL<24>-<23> : op_dpl_lib/Distributed Parameters Line  SimulationMode=ARTEMIS model  Phases=3  Frequency=50  Resistance=[2.619 10.474]/TL_24_23_len  Inductance="[0.111  0.332]/TL_24_23_len"  Capacitance=[0.805e-6 0.365e-6]/TL_24_23_len  Length=TL_24_23_len  Measurements=None
  A24_16 : PMIOPort  Port=1  Side=Left
  B24_16 : PMIOPort  Port=2  Side=Left
  C24_16 : PMIOPort  Port=3  Side=Left
  A21_16 : PMIOPort  Port=4  Side=Left
  B21_16 : PMIOPort  Port=5  Side=Left
  C21_16 : PMIOPort  Port=6  Side=Left
  meas_E sys2 : Outport
  tag scope: GT6_CB=global, GT7_CB=global, load21=global, load23=global, load24=global
  wires:
  Machines Measurements/1(Machines Measurements) -> Mux/1
  Mux/1 -> Memory/1
  Memory/1 -> meas_E sys2/1
  Buses voltages_E/1(Voltages) -> Mux/2
  Buses current_E/1(current) -> Mux/3
  ctrl_E sys2/1 -> OpComm/1
  Demux/1 -> Demux1/1
  Demux/2 -> Demux2/1
  Demux1/2 -> [GT7_CB]
  Demux1/1 -> [GT6_CB]
  Demux2/1 -> [load21]
  Demux2/2 -> [load23]
  Demux2/3 -> [load24]
  OpComm/1 -> Demux/1
  connections:
  Bus 24/RConn3 -- C24_16/RConn1
  Bus 24/RConn2 -- B24_16/RConn1
  Bus 24/RConn1 -- Load Flow Bus7/LConn1 -- A24_16/RConn1
  TL<24>-<23>/RConn3 -- TL<22>-<23>/RConn3 -- Load 23/LConn3 -- Bus 23/RConn3
  Load 23/LConn2 -- TL<22>-<23>/RConn2 -- TL<24>-<23>/RConn2 -- Bus 23/RConn2
  Load 23/LConn1 -- TL<22>-<23>/RConn1 -- TL<24>-<23>/RConn1 -- Bus 23/RConn1
  GT 7/RConn3 -- Bus 23/LConn3 -- Load Flow Bus8/LConn1
  Bus 23/LConn2 -- GT 7/RConn2
  GT 7/RConn1 -- Bus 23/LConn1
  Bus 22/RConn3 -- TL<21>-<22>/RConn3 -- GT 6/RConn3
  GT 6/RConn2 -- TL<21>-<22>/RConn2 -- Bus 22/RConn2
  Load Flow Bus9/LConn1 -- TL<21>-<22>/RConn1 -- GT 6/RConn1 -- Bus 22/RConn1
  TL<22>-<23>/LConn3 -- Bus 22/LConn3
  Bus 22/LConn2 -- TL<22>-<23>/LConn2
  TL<22>-<23>/LConn1 -- Bus 22/LConn1
  Bus 21/RConn1 -- Load 21/LConn1 -- TL<21>-<22>/LConn1
  Bus 21/RConn2 -- Load 21/LConn2 -- TL<21>-<22>/LConn2
  Bus 21/RConn3 -- Load 21/LConn3 -- TL<21>-<22>/LConn3
  C21_16/RConn1 -- Load Flow Bus5/LConn1 -- Bus 21/LConn3
  Load 24/LConn1 -- TL<24>-<23>/LConn1 -- Bus 24/LConn1
  Load 24/LConn2 -- TL<24>-<23>/LConn2 -- Bus 24/LConn2
  Bus 24/LConn3 -- TL<24>-<23>/LConn3 -- Load 24/LConn3
  Bus 21/LConn2 -- B21_16/RConn1
  A21_16/RConn1 -- Bus 21/LConn1

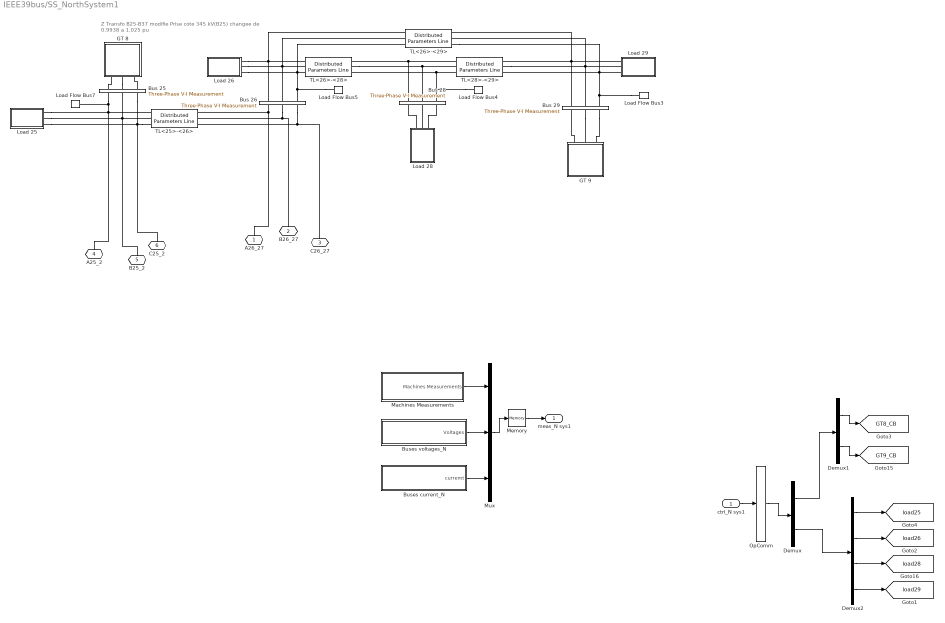
== system IEEE39bus/SS_NorthSystem1 ==
  note: Z Transfo B25-B37 modifie
      | Prise cote 345 kV(B25)  changee de 0.9938 a 1.025 pu
  ctrl_N sys1 : Inport
  Bus 25 : powerlib/Measurements/Three-Phase V-I Measurement  VoltageMeasurement=phase-to-ground  SetLabelV=on  LabelV=V_bus_25  Vpu=off  VpuLL=off  CurrentMeasurement=yes  SetLabelI=on  LabelI=I_bus_25  Ipu=off  Pbase=100e6  Vbase=230e3  OutputType=Complex  PhasorSimulation=off  PSBequivalent=0
  Bus 26 : powerlib/Measurements/Three-Phase V-I Measurement  VoltageMeasurement=phase-to-ground  SetLabelV=on  LabelV=V_bus_26  Vpu=off  VpuLL=off  CurrentMeasurement=yes  SetLabelI=on  LabelI=I_bus_26  Ipu=off  Pbase=100e6  Vbase=230e3  OutputType=Complex  PhasorSimulation=off  PSBequivalent=0
  Bus 28 : powerlib/Measurements/Three-Phase V-I Measurement  VoltageMeasurement=phase-to-ground  SetLabelV=on  LabelV=V_bus_28  Vpu=off  VpuLL=off  CurrentMeasurement=yes  SetLabelI=on  LabelI=I_bus_28  Ipu=off  Pbase=100e6  Vbase=230e3  OutputType=Complex  PhasorSimulation=off  PSBequivalent=0
  Bus 29 : powerlib/Measurements/Three-Phase V-I Measurement  VoltageMeasurement=phase-to-ground  SetLabelV=on  LabelV=V_bus_29  Vpu=off  VpuLL=off  CurrentMeasurement=yes  SetLabelI=on  LabelI=I_bus_29  Ipu=off  Pbase=100e6  Vbase=230e3  OutputType=Complex  PhasorSimulation=off  PSBequivalent=0
  Buses current_N : Subsystem
  Buses voltages_N : Subsystem
  Demux : Demux  Outputs=[2 8]
  Demux1 : Demux  Outputs=2
  Demux2 : Demux  Outputs=[2 2 2 2]
  GT 8 : Subsystem
  GT 9 : Subsystem
  Load 25 : Subsystem  SystemSampleTime=20e-3
  Load 26 : Subsystem  SystemSampleTime=20e-3
  Load 28 : Subsystem  SystemSampleTime=20e-3
  Load 29 : Subsystem  SystemSampleTime=20e-3
  Load Flow Bus3 : powerlib/Measurements/Load Flow Bus  LConnTagsString=a  ID=Bus-29  Vbase=345e+003  Vref=1  Vangle=0  VLF=1.034  angleLF=25.68
      settings: AttributesFormatString=%<ID>\n%<Vbase>V\n%<VLF>pu\n%<angleLF>deg.
  Load Flow Bus4 : powerlib/Measurements/Load Flow Bus  LConnTagsString=a  ID=Bus-28  Vbase=345e+003  Vref=1  Vangle=0  VLF=1.031  angleLF=23.66
      settings: AttributesFormatString=%<ID>\n%<Vbase>V\n%<VLF>pu\n%<angleLF>deg.
  Load Flow Bus5 : powerlib/Measurements/Load Flow Bus  LConnTagsString=a  ID=Bus-26  Vbase=345e+003  Vref=1  Vangle=0  VLF=1.027  angleLF=21.79
      settings: AttributesFormatString=%<ID>\n%<Vbase>V\n%<VLF>pu\n%<angleLF>deg.
  Load Flow Bus7 : powerlib/Measurements/Load Flow Bus  LConnTagsString=a  ID=Bus-25  Vbase=345e+003  Vref=1  Vangle=0  VLF=1.034  angleLF=25.05
      settings: AttributesFormatString=%<ID>\n%<Vbase>V\n%<VLF>pu\n%<angleLF>deg.
  Machines Measurements : Subsystem
      mask Display: disp('Machines Measurements')
  Memory : Memory
  Mux : Mux  Inputs=3
  OpComm : rtlab/OpComm  nbport=1  groupe_acq=1  subsys_rate=0  st=0  Synchronization=on  Interpolation=on  Threshold=1.0  Missed_Data=off  Sim_Time=off  Samples=off  dynSigOut=off  from_console=0  warning_done=off  writeOpCommFile=off  Offset=off
  TL<25>-<26> : op_dpl_lib/Distributed Parameters Line  SimulationMode=ARTEMIS model  Phases=3  Frequency=50  Resistance=[3.809 15.235]/TL_25_26_len  Inductance="[0.102  0.306]/TL_25_26_len"  Capacitance=[1.143e-6 0.52e-6]/TL_25_26_len  Length=TL_25_26_len  Measurements=None
  TL<26>-<28> : op_dpl_lib/Distributed Parameters Line  SimulationMode=ARTEMIS model  Phases=3  Frequency=50  Resistance=[5.118 20.472]/TL_26_28_len  Inductance="[0.15  0.449]/TL_26_28_len"  Capacitance=[1.739e-6 0.791e-6]/TL_26_28_len  Length=TL_26_28_len  Measurements=None
  TL<26>-<29> : op_dpl_lib/Distributed Parameters Line  SimulationMode=ARTEMIS model  Phases=3  Frequency=50  Resistance=[6.784 27.138]/TL_26_29_len  Inductance="[0.197  0.592]/TL_26_29_len"  Capacitance=[2.293e-6 1.043e-6]/TL_26_29_len  Length=TL_26_29_len  Measurements=None
  TL<28>-<29> : op_dpl_lib/Distributed Parameters Line  SimulationMode=ARTEMIS model  Phases=3  Frequency=50  Resistance=[1.666 6.665]/TL_28_29_len  Inductance="[0.048  0.143]/TL_28_29_len"  Capacitance=[0.555e-6 0.252e-6]/TL_28_29_len  Length=TL_28_29_len  Measurements=None
  A26_27 : PMIOPort  Port=1  Side=Left
  B26_27 : PMIOPort  Port=2  Side=Left
  C26_27 : PMIOPort  Port=3  Side=Left
  A25_2 : PMIOPort  Port=4  Side=Left
  B25_2 : PMIOPort  Port=5  Side=Left
  C25_2 : PMIOPort  Port=6  Side=Left
  meas_N sys1 : Outport
  tag scope: GT8_CB=global, GT9_CB=global, load25=global, load26=global, load28=global, load29=global
  wires:
  Machines Measurements/1(Machines Measurements) -> Mux/1
  Mux/1 -> Memory/1
  Memory/1 -> meas_N sys1/1
  Buses voltages_N/1(Voltages) -> Mux/2
  Buses current_N/1(curremt) -> Mux/3
  ctrl_N sys1/1 -> OpComm/1
  OpComm/1 -> Demux/1
  Demux/2 -> Demux2/1
  Demux/1 -> Demux1/1
  Demux1/1 -> [GT8_CB]
  Demux1/2 -> [GT9_CB]
  Demux2/1 -> [load25]
  Demux2/2 -> [load26]
  Demux2/3 -> [load28]
  Demux2/4 -> [load29]
  connections:
  Load Flow Bus3/LConn1 -- Bus 29/RConn3 -- TL<28>-<29>/RConn3 -- Load 29/LConn3 -- TL<26>-<29>/RConn3
  Load 29/LConn2 -- TL<28>-<29>/RConn2 -- TL<26>-<29>/RConn2 -- Bus 29/RConn2
  Bus 29/LConn3 -- GT 9/RConn3
  Bus 29/LConn2 -- GT 9/RConn2
  GT 9/RConn1 -- Bus 29/LConn1
  TL<28>-<29>/LConn2 -- TL<26>-<28>/RConn2 -- Bus 28/RConn2
  Load 28/LConn3 -- Bus 28/LConn3
  Load 28/LConn2 -- Bus 28/LConn2
  Load 28/LConn1 -- Bus 28/LConn1
  Bus 25/RConn3 -- GT 8/RConn3
  GT 8/RConn2 -- Bus 25/RConn2
  GT 8/RConn1 -- Bus 25/RConn1
  TL<25>-<26>/LConn3 -- C25_2/RConn1 -- Load 25/LConn3 -- Bus 25/LConn3
  Load 25/LConn2 -- B25_2/RConn1 -- TL<25>-<26>/LConn2 -- Bus 25/LConn2
  Load Flow Bus7/LConn1 -- Bus 25/LConn1 -- Load 25/LConn1 -- A25_2/RConn1 -- TL<25>-<26>/LConn1
  Load Flow Bus5/LConn1 -- TL<26>-<29>/LConn3 -- Load 26/LConn3 -- TL<26>-<28>/LConn3 -- Bus 26/RConn3
  A26_27/RConn1 -- TL<25>-<26>/RConn1 -- Bus 26/LConn1
  Bus 26/LConn2 -- TL<25>-<26>/RConn2 -- B26_27/RConn1
  Bus 26/LConn3 -- TL<25>-<26>/RConn3 -- C26_27/RConn1
  Load 26/LConn1 -- TL<26>-<29>/LConn1 -- Bus 26/RConn1 -- TL<26>-<28>/LConn1
  Load 26/LConn2 -- TL<26>-<29>/LConn2 -- TL<26>-<28>/LConn2 -- Bus 26/RConn2
  TL<28>-<29>/LConn1 -- TL<26>-<28>/RConn1 -- Bus 28/RConn1
  Load Flow Bus4/LConn1 -- TL<26>-<28>/RConn3 -- TL<28>-<29>/LConn3 -- Bus 28/RConn3
  Load 29/LConn1 -- TL<28>-<29>/RConn1 -- TL<26>-<29>/RConn1 -- Bus 29/RConn1
